simulink model "Step_12_TheEstimatedINVDynamicsMatricesCTC"  (R2020a)
settings: Solver=ode4  StartTime=0.0  StopTime=10  FixedStep=2e-3  RelTol=1e-3
model workspace (MATLAB code in the model file):
  | dhparams = [0   0   0.6   0;
  |             0   0   0     pi/2;
  |             0   0   0.5   0];
  | 
  | rrrRobot = rigidBodyTree('DataFormat', 'column', 'MaxNumBodies', 4);
  | 
  | bodyNames = {'link1', 'link2', 'link3'};
  | jointNames = {'joint1', 'joint2', 'joint3'};
  | parentNames = {'base', 'link1', 'link2'};
  | 
  | for i = 1:3
  |     body = rigidBody(bodyNames{i});
  |     joint = rigidBodyJoint(jointNames{i}, 'revolute');
  |     setFixedTransform(joint, dhparams(i,:), 'dh');
  |     body.Joint = joint;
  |     addBody(rrrRobot, body, parentNames{i});
  | end
  | 
  | tool = rigidBody('tool');
  | jointTool = rigidBodyJoint('fix_tip', 'fixed');
  | setFixedTransform(jointTool, eye(4));
  | tool.Joint = jointTool;
  | addBody(rrrRobot, tool, 'link3');
values from neighbouring files (symbols this model uses):
  N = simplify(N,'Seconds',30)    [Step_1_GetTheRegressorMatrix.m]    (also in Step_1_TheRegressorModel.m)
  s = size(M)    [Step_1_GetTheRegressorMatrix.m]    (also in Step_1_TheRegressorModel.m)
  Y = sym(zeros(robot.nbDOF,numel(Xhi)))    [Step_1_GetTheRegressorMatrix.m]    (also in Step_1_TheRegressorModel.m)
  Z = robot.symbolicParameters.Z    [Step_1_GetTheRegressorMatrix.m]    (also in Step_1_TheRegressorModel.m)
undefined symbols (not defined in the file or in its folder): X
libraries: sm_lib x34, nesl_utility x10
(part 2 of 2)

== matlab function Step_12_TheEstimatedINVDynamicsMatricesCTC/CTC/Estimated_C ==
  data: in1 input; EstTau_C output; in2 input
function EstTau_C = Estimated_C(in1,in2)
%#codegen

%    This function was generated by the Symbolic Math Toolbox version 8.5.
%    15-Jul-2026 04:23:10

q1 = in1(1,:);
q2 = in1(2,:);
q3 = in1(3,:);
qp1 = in2(1,:);
qp2 = in2(2,:);
qp3 = in2(3,:);
EstTau_C = [qp1.*2.995651003090984e-1+tanh(qp1.*1.0e+2).*2.011490037900599e-1+(cos(q2+q3).*cos(q1).*(qp2.*cos(q1)+qp3.*cos(q1))+cos(q2+q3).*sin(q1).*(qp2.*sin(q1)+qp3.*sin(q1))).*(qp1.*sin(q2+q3)-cos(q2+q3).*sin(q1).*(qp2.*cos(q1)+qp3.*cos(q1))+cos(q2+q3).*cos(q1).*(qp2.*sin(q1)+qp3.*sin(q1))).*1.461022037882879e-2+cos(q2+q3).*(sin(q1).*(qp1.*qp2.*cos(q1)+qp1.*qp3.*cos(q1))-cos(q1).*(qp1.*qp2.*sin(q1)+qp1.*qp3.*sin(q1))).*8.257807196549019e-4+(qp2.*cos(q1).^2.*sin(q2)+qp2.*sin(q1).^2.*sin(q2)).*(qp2.*cos(q1).^2+qp2.*sin(q1).^2).*1.019521576964412e-3-(cos(q2+q3).*cos(q1).*(qp2.*cos(q1)+qp3.*cos(q1))+cos(q2+q3).*sin(q1).*(qp2.*sin(q1)+qp3.*sin(q1))).*(qp1.*cos(q2+q3)+sin(q2+q3).*sin(q1).*(qp2.*cos(q1)+qp3.*cos(q1))-sin(q2+q3).*cos(q1).*(qp2.*sin(q1)+qp3.*sin(q1))).*4.225263872871405e-4-sin(q2+q3).*(sin(q1).*(qp1.*qp2.*cos(q1)+qp1.*qp3.*cos(q1))-cos(q1).*(qp1.*qp2.*sin(q1)+qp1.*qp3.*sin(q1))).*4.587581372374521e-4+(sin(q2+q3).*cos(q1).*(qp2.*cos(q1)+qp3.*cos(q1))+sin(q2+q3).*sin(q1).*(qp2.*sin(q1)+qp3.*sin(q1))).*(qp1.*sin(q2+q3)-cos(q2+q3).*sin(q1).*(qp2.*cos(q1)+qp3.*cos(q1))+cos(q2+q3).*cos(q1).*(qp2.*sin(q1)+qp3.*sin(q1))).*4.225263872871405e-4-cos(q2+q3).*((cos(q1).*cos(q2).*(qp1.*qp2.*cos(q1)+qp1.*qp3.*cos(q1)))./2.0+(cos(q2).*sin(q1).*(qp1.*qp2.*sin(q1)+qp1.*qp3.*sin(q1)))./2.0+(qp1.*cos(q1).*cos(q2).*(qp2.*cos(q1)+qp3.*cos(q1)))./2.0+(qp1.*cos(q2).*sin(q1).*(qp2.*sin(q1)+qp3.*sin(q1)))./2.0).*2.255824778756872e-3+cos(q2).*(qp1.*qp2.*cos(q1).^2.*cos(q2)+qp1.*qp2.*cos(q2).*sin(q1).^2).*1.124368820605591e-3-(sin(q2+q3).*cos(q1).*(qp2.*cos(q1)+qp3.*cos(q1))+sin(q2+q3).*sin(q1).*(qp2.*sin(q1)+qp3.*sin(q1))).*(qp1.*cos(q2+q3)+sin(q2+q3).*sin(q1).*(qp2.*cos(q1)+qp3.*cos(q1))-sin(q2+q3).*cos(q1).*(qp2.*sin(q1)+qp3.*sin(q1))).*9.399293254739789e-2-(sin(q1).*(qp2.*sin(q1)+qp3.*sin(q1))+cos(q1).*(qp2.*cos(q1)+qp3.*cos(q1))).*(cos(q2+q3).*cos(q1).*(qp2.*cos(q1)+qp3.*cos(q1))+cos(q2+q3).*sin(q1).*(qp2.*sin(q1)+qp3.*sin(q1))).*4.587581372374521e-4-sin(q2+q3).*((cos(q1).*cos(q2).*(qp1.*qp2.*cos(q1)+qp1.*qp3.*cos(q1)))./2.0+(cos(q2).*sin(q1).*(qp1.*qp2.*sin(q1)+qp1.*qp3.*sin(q1)))./2.0+(qp1.*cos(q1).*cos(q2).*(qp2.*cos(q1)+qp3.*cos(q1)))./2.0+(qp1.*cos(q2).*sin(q1).*(qp2.*sin(q1)+qp3.*sin(q1)))./2.0).*2.999511617512276e-1-cos(q2).*(qp1.*qp2.*cos(q1).^2.*sin(q2)+qp1.*qp2.*sin(q1).^2.*sin(q2)).*5.841025348904085e-1-cos(q2+q3).*(cos(q2+q3).*cos(q1).*(qp1.*qp2.*cos(q1)+qp1.*qp3.*cos(q1))+cos(q2+q3).*sin(q1).*(qp1.*qp2.*sin(q1)+qp1.*qp3.*sin(q1))).*4.225263872871405e-4-(sin(q1).*(qp2.*sin(q1)+qp3.*sin(q1))+cos(q1).*(qp2.*cos(q1)+qp3.*cos(q1))).*(sin(q2+q3).*cos(q1).*(qp2.*cos(q1)+qp3.*cos(q1))+sin(q2+q3).*sin(q1).*(qp2.*sin(q1)+qp3.*sin(q1))).*8.257807196549019e-4-sin(q2).*(qp1.*qp2.*cos(q1).^2.*sin(q2)+qp1.*qp2.*sin(q1).^2.*sin(q2)).*1.124368820605591e-3+sin(q2+q3).*(cos(q2+q3).*cos(q1).*(qp1.*qp2.*cos(q1)+qp1.*qp3.*cos(q1))+cos(q2+q3).*sin(q1).*(qp1.*qp2.*sin(q1)+qp1.*qp3.*sin(q1))).*1.461022037882879e-2-cos(q2+q3).*(sin(q2+q3).*cos(q1).*(qp1.*qp2.*cos(q1)+qp1.*qp3.*cos(q1))+sin(q2+q3).*sin(q1).*(qp1.*qp2.*sin(q1)+qp1.*qp3.*sin(q1))).*9.399293254739789e-2+sin(q2+q3).*(sin(q2+q3).*cos(q1).*(qp1.*qp2.*cos(q1)+qp1.*qp3.*cos(q1))+sin(q2+q3).*sin(q1).*(qp1.*qp2.*sin(q1)+qp1.*qp3.*sin(q1))).*4.225263872871405e-4-(sin(q1).*(qp2.*cos(q1)+qp3.*cos(q1))-cos(q1).*(qp2.*sin(q1)+qp3.*sin(q1))).*(qp1.*sin(q2+q3)-cos(q2+q3).*sin(q1).*(qp2.*cos(q1)+qp3.*cos(q1))+cos(q2+q3).*cos(q1).*(qp2.*sin(q1)+qp3.*sin(q1))).*4.587581372374521e-4+(sin(q1).*(qp2.*cos(q1)+qp3.*cos(q1))-cos(q1).*(qp2.*sin(q1)+qp3.*sin(q1))).*(qp1.*cos(q2+q3)+sin(q2+q3).*sin(q1).*(qp2.*cos(q1)+qp3.*cos(q1))-sin(q2+q3).*cos(q1).*(qp2.*sin(q1)+qp3.*sin(q1))).*8.257807196549019e-4+(sin(q1).*(qp2.*sin(q1)+qp3.*sin(q1))+cos(q1).*(qp2.*cos(q1)+qp3.*cos(q1))).*(sin(q1).*(qp2.*cos(q1)+qp3.*cos(q1))-cos(q1).*(qp2.*sin(q1)+qp3.*sin(q1))).*8.392301883660855e-2+(qp2.*cos(q1).^2.*cos(q2)+qp2.*cos(q2).*sin(q1).^2).*(qp2.*cos(q1).^2+qp2.*sin(q1).^2).*1.026288799911739e-3-cos(q2+q3).*cos(q1).*(qp1.*((qp1.*cos(q2).*sin(q1))./2.0+(qp2.*cos(q1).*sin(q2))./2.0)+qp2.*((qp1.*cos(q1).*sin(q2))./2.0+(qp2.*cos(q2).*sin(q1))./2.0)-(qp2.*cos(q1)+qp3.*cos(q1)).*((cos(q2).*sin(q1).*(qp2.*cos(q1)+qp3.*cos(q1)))./2.0-(cos(q1).*cos(q2).*(qp2.*sin(q1)+qp3.*sin(q1)))./2.0)-(qp1.^2.*cos(q2).*sin(q1))./2.0).*2.999511617512276e-1+sin(q2+q3).*cos(q1).*(qp1.*((qp1.*cos(q2).*sin(q1))./2.0+(qp2.*cos(q1).*sin(q2))./2.0)+qp2.*((qp1.*cos(q1).*sin(q2))./2.0+(qp2.*cos(q2).*sin(q1))./2.0)-(qp2.*cos(q1)+qp3.*cos(q1)).*((cos(q2).*sin(q1).*(qp2.*cos(q1)+qp3.*cos(q1)))./2.0-(cos(q1).*cos(q2).*(qp2.*sin(q1)+qp3.*sin(q1)))./2.0)-(qp1.^2.*cos(q2).*sin(q1))./2.0).*2.255824778756872e-3+cos(q2+q3).*sin(q1).*((qp2.*sin(q1)+qp3.*sin(q1)).*((cos(q2).*sin(q1).*(qp2.*cos(q1)+qp3.*cos(q1)))./2.0-(cos(q1).*cos(q2).*(qp2.*sin(q1)+qp3.*sin(q1)))./2.0)+qp1.*((qp1.*cos(q1).*cos(q2))./2.0-(qp2.*sin(q1).*sin(q2))./2.0)+qp2.*((qp2.*cos(q1).*cos(q2))./2.0-(qp1.*sin(q1).*sin(q2))./2.0)-(qp1.^2.*cos(q1).*cos(q2))./2.0).*2.999511617512276e-1+qp1.*cos(q2).*(qp2.*cos(q1).^2.*cos(q2)+qp2.*cos(q2).*sin(q1).^2).*1.124368820605591e-3-sin(q2+q3).*sin(q1).*((qp2.*sin(q1)+qp3.*sin(q1)).*((cos(q2).*sin(q1).*(qp2.*cos(q1)+qp3.*cos(q1)))./2.0-(cos(q1).*cos(q2).*(qp2.*sin(q1)+qp3.*sin(q1)))./2.0)+qp1.*((qp1.*cos(q1).*cos(q2))./2.0-(qp2.*sin(q1).*sin(q2))./2.0)+qp2.*((qp2.*cos(q1).*cos(q2))./2.0-(qp1.*sin(q1).*sin(q2))./2.0)-(qp1.^2.*cos(q1).*cos(q2))./2.0).*2.255824778756872e-3-qp1.*cos(q2).*(qp2.*cos(q1).^2.*sin(q2)+qp2.*sin(q1).^2.*sin(q2)).*5.841025348904085e-1-qp1.*sin(q2).*(qp2.*cos(q1).^2.*sin(q2)+qp2.*sin(q1).^2.*sin(q2)).*1.124368820605591e-3;qp2.*6.044333007850473e-1+tanh(qp2.*1.0e+2).*4.92616612948365e-1-sin(q1).*((cos(q2+q3).*(qp2.*cos(q1)+qp3.*cos(q1))-qp1.*sin(q2+q3).*sin(q1)).*(qp1.*cos(q2+q3)+sin(q2+q3).*sin(q1).*(qp2.*cos(q1)+qp3.*cos(q1))-sin(q2+q3).*cos(q1).*(qp2.*sin(q1)+qp3.*sin(q1)))-sin(q2+q3).*cos(q1).*(sin(q2+q3).*cos(q1).*(qp1.*qp2.*cos(q1)+qp1.*qp3.*cos(q1))+sin(q2+q3).*sin(q1).*(qp1.*qp2.*sin(q1)+qp1.*qp3.*sin(q1)))).*9.399293254739789e-2-sin(q1).*(-(sin(q1).*(qp2.*sin(q1)+qp3.*sin(q1))+cos(q1).*(qp2.*cos(q1)+qp3.*cos(q1))).*(sin(q2+q3).*(qp2.*cos(q1)+qp3.*cos(q1))+qp1.*cos(q2+q3).*sin(q1))+sin(q1).*(cos(q2+q3).*cos(q1).*(qp1.*qp2.*cos(q1)+qp1.*qp3.*cos(q1))+cos(q2+q3).*sin(q1).*(qp1.*qp2.*sin(q1)+qp1.*qp3.*sin(q1)))+qp1.*cos(q1).*(qp1.*sin(q2+q3)-cos(q2+q3).*sin(q1).*(qp2.*cos(q1)+qp3.*cos(q1))+cos(q2+q3).*cos(q1).*(qp2.*sin(q1)+qp3.*sin(q1)))+cos(q2+q3).*cos(q1).*(sin(q1).*(qp1.*qp2.*cos(q1)+qp1.*qp3.*cos(q1))-cos(q1).*(qp1.*qp2.*sin(q1)+qp1.*qp3.*sin(q1)))).*4.587581372374521e-4-cos(q1).*(-cos(q1).*(qp1.*qp2.*cos(q1).^2.*cos(q2)+qp1.*qp2.*cos(q2).*sin(q1).^2)+(qp1.*cos(q1).*cos(q2)-qp2.*sin(q1).*sin(q2)).*(qp2.*cos(q1).^2+qp2.*sin(q1).^2)+qp1.^2.*sin(q1).*sin(q2)).*1.026288799911739e-3-cos(q2+q3).*((qp2.*sin(q1)+qp3.*sin(q1)).*((cos(q2).*(qp2.*sin(q1)+qp3.*sin(q1)))./2.0+(qp1.*cos(q1).*sin(q2))./2.0)-cos(q1).*(qp1.*((qp1.*cos(q1).*cos(q2))./2.0-(qp2.*sin(q1).*sin(q2))./2.0)+qp2.*((qp2.*cos(q1).*cos(q2))./2.0-(qp1.*sin(q1).*sin(q2))./2.0))-sin(q1).*(qp1.*((qp1.*cos(q2).*sin(q1))./2.0+(qp2.*cos(q1).*sin(q2))./2.0)+qp2.*((qp1.*cos(q1).*sin(q2))./2.0+(qp2.*cos(q2).*sin(q1))./2.0))+(qp2.*cos(q1)+qp3.*cos(q1)).*((cos(q2).*(qp2.*cos(q1)+qp3.*cos(q1)))./2.0-(qp1.*sin(q1).*sin(q2))./2.0)-(sin(q1).*sin(q2).*(qp1.*qp2.*cos(q1)+qp1.*qp3.*cos(q1)))./2.0+(cos(q1).*sin(q2).*(qp1.*qp2.*sin(q1)+qp1.*qp3.*sin(q1)))./2.0).*2.255824778756872e-3+cos(q1).*((cos(q2+q3).*(qp2.*sin(q1)+qp3.*sin(q1))+qp1.*sin(q2+q3).*cos(q1)).*(qp1.*cos(q2+q3)+sin(q2+q3).*sin(q1).*(qp2.*cos(q1)+qp3.*cos(q1))-sin(q2+q3).*cos(q1).*(qp2.*sin(q1)+qp3.*sin(q1)))-sin(q2+q3).*sin(q1).*(sin(q2+q3).*cos(q1).*(qp1.*qp2.*cos(q1)+qp1.*qp3.*cos(q1))+sin(q2+q3).*sin(q1).*(qp1.*qp2.*sin(q1)+qp1.*qp3.*sin(q1)))).*9.399293254739789e-2-cos(q1).*((sin(q1).*(qp2.*sin(q1)+qp3.*sin(q1))+cos(q1).*(qp2.*cos(q1)+qp3.*cos(q1))).*(sin(q2+q3).*(qp2.*sin(q1)+qp3.*sin(q1))-qp1.*cos(q2+q3).*cos(q1))+cos(q1).*(cos(q2+q3).*cos(q1).*(qp1.*qp2.*cos(q1)+qp1.*qp3.*cos(q1))+cos(q2+q3).*sin(q1).*(qp1.*qp2.*sin(q1)+qp1.*qp3.*sin(q1)))-qp1.*sin(q1).*(qp1.*sin(q2+q3)-cos(q2+q3).*sin(q1).*(qp2.*cos(q1)+qp3.*cos(q1))+cos(q2+q3).*cos(q1).*(qp2.*sin(q1)+qp3.*sin(q1)))-cos(q2+q3).*sin(q1).*(sin(q1).*(qp1.*qp2.*cos(q1)+qp1.*qp3.*cos(q1))-cos(q1).*(qp1.*qp2.*sin(q1)+qp1.*qp3.*sin(q1)))).*4.587581372374521e-4+cos(q1).*(-(qp1.*cos(q1).*sin(q2)+qp2.*cos(q2).*sin(q1)).*(qp2.*cos(q1).^2+qp2.*sin(q1).^2)+cos(q1).*(qp1.*qp2.*cos(q1).^2.*sin(q2)+qp1.*qp2.*sin(q1).^2.*sin(q2))+qp1.^2.*cos(q2).*sin(q1)).*1.019521576964412e-3+sin(q1).*(sin(q1).*(qp1.*qp2.*cos(q1).^2.*cos(q2)+qp1.*qp2.*cos(q2).*sin(q1).^2)-(qp1.*cos(q2).*sin(q1)+qp2.*cos(q1).*sin(q2)).*(qp2.*cos(q1).^2+qp2.*sin(q1).^2)+qp1.^2.*cos(q1).*sin(q2)).*1.026288799911739e-3-sin(q2+q3).*((qp2.*sin(q1)+qp3.*sin(q1)).*((cos(q2).*(qp2.*sin(q1)+qp3.*sin(q1)))./2.0+(qp1.*cos(q1).*sin(q2))./2.0)-cos(q1).*(qp1.*((qp1.*cos(q1).*cos(q2))./2.0-(qp2.*sin(q1).*sin(q2))./2.0)+qp2.*((qp2.*cos(q1).*cos(q2))./2.0-(qp1.*sin(q1).*sin(q2))./2.0))-sin(q1).*(qp1.*((qp1.*cos(q2).*sin(q1))./2.0+(qp2.*cos(q1).*sin(q2))./2.0)+qp2.*((qp1.*cos(q1).*sin(q2))./2.0+(qp2.*cos(q2).*sin(q1))./2.0))+(qp2.*cos(q1)+qp3.*cos(q1)).*((cos(q2).*(qp2.*cos(q1)+qp3.*cos(q1)))./2.0-(qp1.*sin(q1).*sin(q2))./2.0)-(sin(q1).*sin(q2).*(qp1.*qp2.*cos(q1)+qp1.*qp3.*cos(q1)))./2.0+(cos(q1).*sin(q2).*(qp1.*qp2.*sin(q1)+qp1.*qp3.*sin(q1)))./2.0).*2.999511617512276e-1-sin(q1).*(qp1.*cos(q2).*(qp1.*cos(q2).*sin(q1)+qp2.*cos(q1).*sin(q2))+cos(q1).*sin(q2).*(qp1.*qp2.*cos(q1).^2.*cos(q2)+qp1.*qp2.*cos(q2).*sin(q1).^2)+qp1.*sin(q2).*(qp2.*cos(q1).*cos(q2)-qp1.*sin(q1).*sin(q2))+cos(q1).*cos(q2).*(qp1.*qp2.*cos(q1).^2.*sin(q2)+qp1.*qp2.*sin(q1).^2.*sin(q2))).*1.124368820605591e-3+sin(q1).*((sin(q2+q3).*(qp2.*cos(q1)+qp3.*cos(q1))+qp1.*cos(q2+q3).*sin(q1)).*(qp1.*cos(q2+q3)+sin(q2+q3).*sin(q1).*(qp2.*cos(q1)+qp3.*cos(q1))-sin(q2+q3).*cos(q1).*(qp2.*sin(q1)+qp3.*sin(q1)))+(cos(q2+q3).*(qp2.*cos(q1)+qp3.*cos(q1))-qp1.*sin(q2+q3).*sin(q1)).*(qp1.*sin(q2+q3)-cos(q2+q3).*sin(q1).*(qp2.*cos(q1)+qp3.*cos(q1))+cos(q2+q3).*cos(q1).*(qp2.*sin(q1)+qp3.*sin(q1)))+sin(q2+q3).*cos(q1).*(cos(q2+q3).*cos(q1).*(qp1.*qp2.*cos(q1)+qp1.*qp3.*cos(q1))+cos(q2+q3).*sin(q1).*(qp1.*qp2.*sin(q1)+qp1.*qp3.*sin(q1)))+cos(q2+q3).*cos(q1).*(sin(q2+q3).*cos(q1).*(qp1.*qp2.*cos(q1)+qp1.*qp3.*cos(q1))+sin(q2+q3).*sin(q1).*(qp1.*qp2.*sin(q1)+qp1.*qp3.*sin(q1)))).*4.225263872871405e-4+sin(q1).*((qp2.*cos(q1).*cos(q2)-qp1.*sin(q1).*sin(q2)).*(qp2.*cos(q1).^2+qp2.*sin(q1).^2)+sin(q1).*(qp1.*qp2.*cos(q1).^2.*sin(q2)+qp1.*qp2.*sin(q1).^2.*sin(q2))-qp1.^2.*cos(q1).*cos(q2)).*1.019521576964412e-3+cos(q2+q3).*cos(q1).^2.*2.93952138516203+cos(q1).*(-qp1.*cos(q2).*(qp1.*cos(q1).*cos(q2)-qp2.*sin(q1).*sin(q2))+qp1.*sin(q2).*(qp1.*cos(q1).*sin(q2)+qp2.*cos(q2).*sin(q1))+sin(q1).*sin(q2).*(qp1.*qp2.*cos(q1).^2.*cos(q2)+qp1.*qp2.*cos(q2).*sin(q1).^2)+cos(q2).*sin(q1).*(qp1.*qp2.*cos(q1).^2.*sin(q2)+qp1.*qp2.*sin(q1).^2.*sin(q2))).*1.124368820605591e-3+cos(q2+q3).*sin(q1).^2.*2.93952138516203-sin(q2+q3).*cos(q1).^2.*2.210708283181735e-2-sin(q1).*((sin(q1).*(qp2.*sin(q1)+qp3.*sin(q1))+cos(q1).*(qp2.*cos(q1)+qp3.*cos(q1))).*(cos(q2+q3).*(qp2.*cos(q1)+qp3.*cos(q1))-qp1.*sin(q2+q3).*sin(q1))+sin(q1).*(sin(q2+q3).*cos(q1).*(qp1.*qp2.*cos(q1)+qp1.*qp3.*cos(q1))+sin(q2+q3).*sin(q1).*(qp1.*qp2.*sin(q1)+qp1.*qp3.*sin(q1)))-qp1.*cos(q1).*(qp1.*cos(q2+q3)+sin(q2+q3).*sin(q1).*(qp2.*cos(q1)+qp3.*cos(q1))-sin(q2+q3).*cos(q1).*(qp2.*sin(q1)+qp3.*sin(q1)))+sin(q2+q3).*cos(q1).*(sin(q1).*(qp1.*qp2.*cos(q1)+qp1.*qp3.*cos(q1))-cos(q1).*(qp1.*qp2.*sin(q1)+qp1.*qp3.*sin(q1)))).*8.257807196549019e-4-sin(q2+q3).*sin(q1).^2.*2.210708283181735e-2+cos(q1).*((sin(q1).*(qp2.*sin(q1)+qp3.*sin(q1))+cos(q1).*(qp2.*cos(q1)+qp3.*cos(q1))).*(cos(q2+q3).*(qp2.*sin(q1)+qp3.*sin(q1))+qp1.*sin(q2+q3).*cos(q1))-cos(q1).*(sin(q2+q3).*cos(q1).*(qp1.*qp2.*cos(q1)+qp1.*qp3.*cos(q1))+sin(q2+q3).*sin(q1).*(qp1.*qp2.*sin(q1)+qp1.*qp3.*sin(q1)))+sin(q2+q3).*sin(q1).*(sin(q1).*(qp1.*qp2.*cos(q1)+qp1.*qp3.*cos(q1))-cos(q1).*(qp1.*qp2.*sin(q1)+qp1.*qp3.*sin(q1)))-qp1.*sin(q1).*(qp1.*cos(q2+q3)+sin(q2+q3).*sin(q1).*(qp2.*cos(q1)+qp3.*cos(q1))-sin(q2+q3).*cos(q1).*(qp2.*sin(q1)+qp3.*sin(q1)))).*8.257807196549019e-4-cos(q1).*((cos(q2+q3).*(qp2.*sin(q1)+qp3.*sin(q1))+qp1.*sin(q2+q3).*cos(q1)).*(qp1.*sin(q2+q3)-cos(q2+q3).*sin(q1).*(qp2.*cos(q1)+qp3.*cos(q1))+cos(q2+q3).*cos(q1).*(qp2.*sin(q1)+qp3.*sin(q1)))+(sin(q2+q3).*(qp2.*sin(q1)+qp3.*sin(q1))-qp1.*cos(q2+q3).*cos(q1)).*(qp1.*cos(q2+q3)+sin(q2+q3).*sin(q1).*(qp2.*cos(q1)+qp3.*cos(q1))-sin(q2+q3).*cos(q1).*(qp2.*sin(q1)+qp3.*sin(q1)))+sin(q2+q3).*sin(q1).*(cos(q2+q3).*cos(q1).*(qp1.*qp2.*cos(q1)+qp1.*qp3.*cos(q1))+cos(q2+q3).*sin(q1).*(qp1.*qp2.*sin(q1)+qp1.*qp3.*sin(q1)))+cos(q2+q3).*sin(q1).*(sin(q2+q3).*cos(q1).*(qp1.*qp2.*cos(q1)+qp1.*qp3.*cos(q1))+sin(q2+q3).*sin(q1).*(qp1.*qp2.*sin(q1)+qp1.*qp3.*sin(q1)))).*4.225263872871405e-4-sin(q1).*((sin(q2+q3).*(qp2.*cos(q1)+qp3.*cos(q1))+qp1.*cos(q2+q3).*sin(q1)).*(qp1.*sin(q2+q3)-cos(q2+q3).*sin(q1).*(qp2.*cos(q1)+qp3.*cos(q1))+cos(q2+q3).*cos(q1).*(qp2.*sin(q1)+qp3.*sin(q1)))-cos(q2+q3).*cos(q1).*(cos(q2+q3).*cos(q1).*(qp1.*qp2.*cos(q1)+qp1.*qp3.*cos(q1))+cos(q2+q3).*sin(q1).*(qp1.*qp2.*sin(q1)+qp1.*qp3.*sin(q1)))).*1.461022037882879e-2+cos(q1).*(cos(q1).*(sin(q1).*(qp1.*qp2.*cos(q1)+qp1.*qp3.*cos(q1))-cos(q1).*(qp1.*qp2.*sin(q1)+qp1.*qp3.*sin(q1)))-qp1.*sin(q1).*(sin(q1).*(qp2.*sin(q1)+qp3.*sin(q1))+cos(q1).*(qp2.*cos(q1)+qp3.*cos(q1)))).*8.392301883660855e-2+cos(q1).*((sin(q2+q3).*(qp2.*sin(q1)+qp3.*sin(q1))-qp1.*cos(q2+q3).*cos(q1)).*(qp1.*sin(q2+q3)-cos(q2+q3).*sin(q1).*(qp2.*cos(q1)+qp3.*cos(q1))+cos(q2+q3).*cos(q1).*(qp2.*sin(q1)+qp3.*sin(q1)))-cos(q2+q3).*sin(q1).*(cos(q2+q3).*cos(q1).*(qp1.*qp2.*cos(q1)+qp1.*qp3.*cos(q1))+cos(q2+q3).*sin(q1).*(qp1.*qp2.*sin(q1)+qp1.*qp3.*sin(q1)))).*1.461022037882879e-2+sin(q1).*(sin(q1).*(sin(q1).*(qp1.*qp2.*cos(q1)+qp1.*qp3.*cos(q1))-cos(q1).*(qp1.*qp2.*sin(q1)+qp1.*qp3.*sin(q1)))+qp1.*cos(q1).*(sin(q1).*(qp2.*sin(q1)+qp3.*sin(q1))+cos(q1).*(qp2.*cos(q1)+qp3.*cos(q1)))).*8.392301883660855e-2+cos(q1).*(qp1.*cos(q2).*(qp1.*cos(q1).*sin(q2)+qp2.*cos(q2).*sin(q1))-sin(q1).*sin(q2).*(qp1.*qp2.*cos(q1).^2.*sin(q2)+qp1.*qp2.*sin(q1).^2.*sin(q2))).*5.841025348904085e-1-sin(q1).*(qp1.*cos(q2).*(qp2.*cos(q1).*cos(q2)-qp1.*sin(q1).*sin(q2))-cos(q1).*sin(q2).*(qp1.*qp2.*cos(q1).^2.*sin(q2)+qp1.*qp2.*sin(q1).^2.*sin(q2))).*5.841025348904085e-1+cos(q2+q3).*cos(q1).*(((cos(q1).*sin(q2).*(qp2.*cos(q1)+qp3.*cos(q1)))./2.0+(sin(q1).*sin(q2).*(qp2.*sin(q1)+qp3.*sin(q1)))./2.0).*(qp2.*cos(q1)+qp3.*cos(q1))-cos(q1).*((qp2.^2.*sin(q2))./2.0+4.9e+1./5.0)+qp1.*((cos(q2).*(qp2.*sin(q1)+qp3.*sin(q1)))./2.0+(qp1.*cos(q1).*sin(q2))./2.0)-(cos(q2).*(qp1.*qp2.*sin(q1)+qp1.*qp3.*sin(q1)))./2.0).*2.999511617512276e-1-sin(q2+q3).*cos(q1).*(((cos(q1).*sin(q2).*(qp2.*cos(q1)+qp3.*cos(q1)))./2.0+(sin(q1).*sin(q2).*(qp2.*sin(q1)+qp3.*sin(q1)))./2.0).*(qp2.*cos(q1)+qp3.*cos(q1))-cos(q1).*((qp2.^2.*sin(q2))./2.0+4.9e+1./5.0)+qp1.*((cos(q2).*(qp2.*sin(q1)+qp3.*sin(q1)))./2.0+(qp1.*cos(q1).*sin(q2))./2.0)-(cos(q2).*(qp1.*qp2.*sin(q1)+qp1.*qp3.*sin(q1)))./2.0).*2.255824778756872e-3+cos(q2+q3).*sin(q1).*(((cos(q1).*sin(q2).*(qp2.*cos(q1)+qp3.*cos(q1)))./2.0+(sin(q1).*sin(q2).*(qp2.*sin(q1)+qp3.*sin(q1)))./2.0).*(qp2.*sin(q1)+qp3.*sin(q1))-qp1.*((cos(q2).*(qp2.*cos(q1)+qp3.*cos(q1)))./2.0-(qp1.*sin(q1).*sin(q2))./2.0)-sin(q1).*((qp2.^2.*sin(q2))./2.0+4.9e+1./5.0)+(cos(q2).*(qp1.*qp2.*cos(q1)+qp1.*qp3.*cos(q1)))./2.0).*2.999511617512276e-1-sin(q2+q3).*sin(q1).*(((cos(q1).*sin(q2).*(qp2.*cos(q1)+qp3.*cos(q1)))./2.0+(sin(q1).*sin(q2).*(qp2.*sin(q1)+qp3.*sin(q1)))./2.0).*(qp2.*sin(q1)+qp3.*sin(q1))-qp1.*((cos(q2).*(qp2.*cos(q1)+qp3.*cos(q1)))./2.0-(qp1.*sin(q1).*sin(q2))./2.0)-sin(q1).*((qp2.^2.*sin(q2))./2.0+4.9e+1./5.0)+(cos(q2).*(qp1.*qp2.*cos(q1)+qp1.*qp3.*cos(q1)))./2.0).*2.255824778756872e-3;qp3.*5.444152870511105e-1+tanh(qp3.*1.0e+2).*7.756228967740465e-1-sin(q1).*((cos(q2+q3).*(qp2.*cos(q1)+qp3.*cos(q1))-qp1.*sin(q2+q3).*sin(q1)).*(qp1.*cos(q2+q3)+sin(q2+q3).*sin(q1).*(qp2.*cos(q1)+qp3.*cos(q1))-sin(q2+q3).*cos(q1).*(qp2.*sin(q1)+qp3.*sin(q1)))-sin(q2+q3).*cos(q1).*(sin(q2+q3).*cos(q1).*(qp1.*qp2.*cos(q1)+qp1.*qp3.*cos(q1))+sin(q2+q3).*sin(q1).*(qp1.*qp2.*sin(q1)+qp1.*qp3.*sin(q1)))).*9.399293254739789e-2-sin(q1).*(-(sin(q1).*(qp2.*sin(q1)+qp3.*sin(q1))+cos(q1).*(qp2.*cos(q1)+qp3.*cos(q1))).*(sin(q2+q3).*(qp2.*cos(q1)+qp3.*cos(q1))+qp1.*cos(q2+q3).*sin(q1))+sin(q1).*(cos(q2+q3).*cos(q1).*(qp1.*qp2.*cos(q1)+qp1.*qp3.*cos(q1))+cos(q2+q3).*sin(q1).*(qp1.*qp2.*sin(q1)+qp1.*qp3.*sin(q1)))+qp1.*cos(q1).*(qp1.*sin(q2+q3)-cos(q2+q3).*sin(q1).*(qp2.*cos(q1)+qp3.*cos(q1))+cos(q2+q3).*cos(q1).*(qp2.*sin(q1)+qp3.*sin(q1)))+cos(q2+q3).*cos(q1).*(sin(q1).*(qp1.*qp2.*cos(q1)+qp1.*qp3.*cos(q1))-cos(q1).*(qp1.*qp2.*sin(q1)+qp1.*qp3.*sin(q1)))).*4.587581372374521e-4+cos(q1).*((cos(q2+q3).*(qp2.*sin(q1)+qp3.*sin(q1))+qp1.*sin(q2+q3).*cos(q1)).*(qp1.*cos(q2+q3)+sin(q2+q3).*sin(q1).*(qp2.*cos(q1)+qp3.*cos(q1))-sin(q2+q3).*cos(q1).*(qp2.*sin(q1)+qp3.*sin(q1)))-sin(q2+q3).*sin(q1).*(sin(q2+q3).*cos(q1).*(qp1.*qp2.*cos(q1)+qp1.*qp3.*cos(q1))+sin(q2+q3).*sin(q1).*(qp1.*qp2.*sin(q1)+qp1.*qp3.*sin(q1)))).*9.399293254739789e-2-cos(q1).*((sin(q1).*(qp2.*sin(q1)+qp3.*sin(q1))+cos(q1).*(qp2.*cos(q1)+qp3.*cos(q1))).*(sin(q2+q3).*(qp2.*sin(q1)+qp3.*sin(q1))-qp1.*cos(q2+q3).*cos(q1))+cos(q1).*(cos(q2+q3).*cos(q1).*(qp1.*qp2.*cos(q1)+qp1.*qp3.*cos(q1))+cos(q2+q3).*sin(q1).*(qp1.*qp2.*sin(q1)+qp1.*qp3.*sin(q1)))-qp1.*sin(q1).*(qp1.*sin(q2+q3)-cos(q2+q3).*sin(q1).*(qp2.*cos(q1)+qp3.*cos(q1))+cos(q2+q3).*cos(q1).*(qp2.*sin(q1)+qp3.*sin(q1)))-cos(q2+q3).*sin(q1).*(sin(q1).*(qp1.*qp2.*cos(q1)+qp1.*qp3.*cos(q1))-cos(q1).*(qp1.*qp2.*sin(q1)+qp1.*qp3.*sin(q1)))).*4.587581372374521e-4+sin(q1).*((sin(q2+q3).*(qp2.*cos(q1)+qp3.*cos(q1))+qp1.*cos(q2+q3).*sin(q1)).*(qp1.*cos(q2+q3)+sin(q2+q3).*sin(q1).*(qp2.*cos(q1)+qp3.*cos(q1))-sin(q2+q3).*cos(q1).*(qp2.*sin(q1)+qp3.*sin(q1)))+(cos(q2+q3).*(qp2.*cos(q1)+qp3.*cos(q1))-qp1.*sin(q2+q3).*sin(q1)).*(qp1.*sin(q2+q3)-cos(q2+q3).*sin(q1).*(qp2.*cos(q1)+qp3.*cos(q1))+cos(q2+q3).*cos(q1).*(qp2.*sin(q1)+qp3.*sin(q1)))+sin(q2+q3).*cos(q1).*(cos(q2+q3).*cos(q1).*(qp1.*qp2.*cos(q1)+qp1.*qp3.*cos(q1))+cos(q2+q3).*sin(q1).*(qp1.*qp2.*sin(q1)+qp1.*qp3.*sin(q1)))+cos(q2+q3).*cos(q1).*(sin(q2+q3).*cos(q1).*(qp1.*qp2.*cos(q1)+qp1.*qp3.*cos(q1))+sin(q2+q3).*sin(q1).*(qp1.*qp2.*sin(q1)+qp1.*qp3.*sin(q1)))).*4.225263872871405e-4+cos(q2+q3).*cos(q1).^2.*2.93952138516203+cos(q2+q3).*sin(q1).^2.*2.93952138516203-sin(q2+q3).*cos(q1).^2.*2.210708283181735e-2-sin(q1).*((sin(q1).*(qp2.*sin(q1)+qp3.*sin(q1))+cos(q1).*(qp2.*cos(q1)+qp3.*cos(q1))).*(cos(q2+q3).*(qp2.*cos(q1)+qp3.*cos(q1))-qp1.*sin(q2+q3).*sin(q1))+sin(q1).*(sin(q2+q3).*cos(q1).*(qp1.*qp2.*cos(q1)+qp1.*qp3.*cos(q1))+sin(q2+q3).*sin(q1).*(qp1.*qp2.*sin(q1)+qp1.*qp3.*sin(q1)))-qp1.*cos(q1).*(qp1.*cos(q2+q3)+sin(q2+q3).*sin(q1).*(qp2.*cos(q1)+qp3.*cos(q1))-sin(q2+q3).*cos(q1).*(qp2.*sin(q1)+qp3.*sin(q1)))+sin(q2+q3).*cos(q1).*(sin(q1).*(qp1.*qp2.*cos(q1)+qp1.*qp3.*cos(q1))-cos(q1).*(qp1.*qp2.*sin(q1)+qp1.*qp3.*sin(q1)))).*8.257807196549019e-4-sin(q2+q3).*sin(q1).^2.*2.210708283181735e-2+cos(q1).*((sin(q1).*(qp2.*sin(q1)+qp3.*sin(q1))+cos(q1).*(qp2.*cos(q1)+qp3.*cos(q1))).*(cos(q2+q3).*(qp2.*sin(q1)+qp3.*sin(q1))+qp1.*sin(q2+q3).*cos(q1))-cos(q1).*(sin(q2+q3).*cos(q1).*(qp1.*qp2.*cos(q1)+qp1.*qp3.*cos(q1))+sin(q2+q3).*sin(q1).*(qp1.*qp2.*sin(q1)+qp1.*qp3.*sin(q1)))+sin(q2+q3).*sin(q1).*(sin(q1).*(qp1.*qp2.*cos(q1)+qp1.*qp3.*cos(q1))-cos(q1).*(qp1.*qp2.*sin(q1)+qp1.*qp3.*sin(q1)))-qp1.*sin(q1).*(qp1.*cos(q2+q3)+sin(q2+q3).*sin(q1).*(qp2.*cos(q1)+qp3.*cos(q1))-sin(q2+q3).*cos(q1).*(qp2.*sin(q1)+qp3.*sin(q1)))).*8.257807196549019e-4-cos(q1).*((cos(q2+q3).*(qp2.*sin(q1)+qp3.*sin(q1))+qp1.*sin(q2+q3).*cos(q1)).*(qp1.*sin(q2+q3)-cos(q2+q3).*sin(q1).*(qp2.*cos(q1)+qp3.*cos(q1))+cos(q2+q3).*cos(q1).*(qp2.*sin(q1)+qp3.*sin(q1)))+(sin(q2+q3).*(qp2.*sin(q1)+qp3.*sin(q1))-qp1.*cos(q2+q3).*cos(q1)).*(qp1.*cos(q2+q3)+sin(q2+q3).*sin(q1).*(qp2.*cos(q1)+qp3.*cos(q1))-sin(q2+q3).*cos(q1).*(qp2.*sin(q1)+qp3.*sin(q1)))+sin(q2+q3).*sin(q1).*(cos(q2+q3).*cos(q1).*(qp1.*qp2.*cos(q1)+qp1.*qp3.*cos(q1))+cos(q2+q3).*sin(q1).*(qp1.*qp2.*sin(q1)+qp1.*qp3.*sin(q1)))+cos(q2+q3).*sin(q1).*(sin(q2+q3).*cos(q1).*(qp1.*qp2.*cos(q1)+qp1.*qp3.*cos(q1))+sin(q2+q3).*sin(q1).*(qp1.*qp2.*sin(q1)+qp1.*qp3.*sin(q1)))).*4.225263872871405e-4+cos(q2+q3).*(cos(q1).*(qp1.*((qp1.*cos(q1).*cos(q2))./2.0-(qp2.*sin(q1).*sin(q2))./2.0)+qp2.*((qp2.*cos(q1).*cos(q2))./2.0-(qp1.*sin(q1).*sin(q2))./2.0))+sin(q1).*(qp1.*((qp1.*cos(q2).*sin(q1))./2.0+(qp2.*cos(q1).*sin(q2))./2.0)+qp2.*((qp1.*cos(q1).*sin(q2))./2.0+(qp2.*cos(q2).*sin(q1))./2.0))).*2.255824778756872e-3+sin(q2+q3).*(cos(q1).*(qp1.*((qp1.*cos(q1).*cos(q2))./2.0-(qp2.*sin(q1).*sin(q2))./2.0)+qp2.*((qp2.*cos(q1).*cos(q2))./2.0-(qp1.*sin(q1).*sin(q2))./2.0))+sin(q1).*(qp1.*((qp1.*cos(q2).*sin(q1))./2.0+(qp2.*cos(q1).*sin(q2))./2.0)+qp2.*((qp1.*cos(q1).*sin(q2))./2.0+(qp2.*cos(q2).*sin(q1))./2.0))).*2.999511617512276e-1-sin(q1).*((sin(q2+q3).*(qp2.*cos(q1)+qp3.*cos(q1))+qp1.*cos(q2+q3).*sin(q1)).*(qp1.*sin(q2+q3)-cos(q2+q3).*sin(q1).*(qp2.*cos(q1)+qp3.*cos(q1))+cos(q2+q3).*cos(q1).*(qp2.*sin(q1)+qp3.*sin(q1)))-cos(q2+q3).*cos(q1).*(cos(q2+q3).*cos(q1).*(qp1.*qp2.*cos(q1)+qp1.*qp3.*cos(q1))+cos(q2+q3).*sin(q1).*(qp1.*qp2.*sin(q1)+qp1.*qp3.*sin(q1)))).*1.461022037882879e-2+cos(q1).*(cos(q1).*(sin(q1).*(qp1.*qp2.*cos(q1)+qp1.*qp3.*cos(q1))-cos(q1).*(qp1.*qp2.*sin(q1)+qp1.*qp3.*sin(q1)))-qp1.*sin(q1).*(sin(q1).*(qp2.*sin(q1)+qp3.*sin(q1))+cos(q1).*(qp2.*cos(q1)+qp3.*cos(q1)))).*8.392301883660855e-2+cos(q1).*((sin(q2+q3).*(qp2.*sin(q1)+qp3.*sin(q1))-qp1.*cos(q2+q3).*cos(q1)).*(qp1.*sin(q2+q3)-cos(q2+q3).*sin(q1).*(qp2.*cos(q1)+qp3.*cos(q1))+cos(q2+q3).*cos(q1).*(qp2.*sin(q1)+qp3.*sin(q1)))-cos(q2+q3).*sin(q1).*(cos(q2+q3).*cos(q1).*(qp1.*qp2.*cos(q1)+qp1.*qp3.*cos(q1))+cos(q2+q3).*sin(q1).*(qp1.*qp2.*sin(q1)+qp1.*qp3.*sin(q1)))).*1.461022037882879e-2+sin(q1).*(sin(q1).*(sin(q1).*(qp1.*qp2.*cos(q1)+qp1.*qp3.*cos(q1))-cos(q1).*(qp1.*qp2.*sin(q1)+qp1.*qp3.*sin(q1)))+qp1.*cos(q1).*(sin(q1).*(qp2.*sin(q1)+qp3.*sin(q1))+cos(q1).*(qp2.*cos(q1)+qp3.*cos(q1)))).*8.392301883660855e-2-cos(q2+q3).*cos(q1).^2.*((qp2.^2.*sin(q2))./2.0+4.9e+1./5.0).*2.999511617512276e-1-cos(q2+q3).*sin(q1).^2.*((qp2.^2.*sin(q2))./2.0+4.9e+1./5.0).*2.999511617512276e-1+sin(q2+q3).*cos(q1).^2.*((qp2.^2.*sin(q2))./2.0+4.9e+1./5.0).*2.255824778756872e-3+sin(q2+q3).*sin(q1).^2.*((qp2.^2.*sin(q2))./2.0+4.9e+1./5.0).*2.255824778756872e-3];

== matlab function Step_12_TheEstimatedINVDynamicsMatricesCTC/CTC/Estimated_G ==
  data: in1 input; EstTau_G output
function EstTau_G = Estimated_G(in1)
%#codegen

%    This function was generated by the Symbolic Math Toolbox version 8.5.
%    15-Jul-2026 04:23:10

q1 = in1(1,:);
q2 = in1(2,:);
q3 = in1(3,:);
EstTau_G = [0.0;cos(q2+q3).*cos(q1).^2.*(-2.93952138516203)-cos(q2+q3).*sin(q1).^2.*2.93952138516203+sin(q2+q3).*cos(q1).^2.*2.210708283181735e-2+sin(q2+q3).*sin(q1).^2.*2.210708283181735e-2-cos(q1).^2.*cos(q2).*1.348620116356317e+1-cos(q2).*sin(q1).^2.*1.348620116356317e+1+cos(q1).^2.*sin(q2).*3.617991560015852e-3+sin(q1).^2.*sin(q2).*3.617991560015852e-3;cos(q2+q3).*cos(q1).^2.*(-2.93952138516203)-cos(q2+q3).*sin(q1).^2.*2.93952138516203+sin(q2+q3).*cos(q1).^2.*2.210708283181735e-2+sin(q2+q3).*sin(q1).^2.*2.210708283181735e-2];

== matlab function Step_12_TheEstimatedINVDynamicsMatricesCTC/CTC/Estimated_M ==
  data: in1 input; EstTau_M output
function EstTau_M = Estimated_M(in1)
%#codegen

%    This function was generated by the Symbolic Math Toolbox version 8.5.
%    15-Jul-2026 04:23:10

q1 = in1(1,:);
q2 = in1(2,:);
q3 = in1(3,:);
EstTau_M = reshape([cos(q2+q3).^2.*9.399293254739789e-2+sin(q2+q3).^2.*1.461022037882879e-2+cos(q2).*sin(q2).*2.248737641211183e-3+cos(q2).^2.*5.841025348904085e-1-cos(q2+q3).*sin(q2+q3).*8.450527745742809e-4+cos(q2+q3).*cos(q1).^2.*cos(q2).*2.999511617512276e-1+cos(q2+q3).*cos(q2).*sin(q1).^2.*2.999511617512276e-1-sin(q2+q3).*cos(q1).^2.*cos(q2).*2.255824778756872e-3-sin(q2+q3).*cos(q2).*sin(q1).^2.*2.255824778756872e-3,sin(q1).*(cos(q2+q3).^2.*cos(q1)-sin(q2+q3).^2.*cos(q1)).*(-4.225263872871405e-4)+cos(q1).*(cos(q2+q3).^2.*sin(q1)-sin(q2+q3).^2.*sin(q1)).*4.225263872871405e-4+cos(q2+q3).*cos(q1).^2.*8.257807196549019e-4+cos(q2+q3).*sin(q1).^2.*8.257807196549019e-4-sin(q2+q3).*cos(q1).^2.*4.587581372374521e-4-sin(q2+q3).*sin(q1).^2.*4.587581372374521e-4-cos(q1).^2.*cos(q2).*1.019521576964412e-3-cos(q2).*sin(q1).^2.*1.019521576964412e-3+cos(q1).^2.*sin(q2).*1.026288799911739e-3+sin(q1).*(cos(q1).*cos(q2).^2-cos(q1).*sin(q2).^2).*1.124368820605591e-3+sin(q1).^2.*sin(q2).*1.026288799911739e-3-cos(q1).*(cos(q2).^2.*sin(q1)-sin(q1).*sin(q2).^2).*1.124368820605591e-3,sin(q1).*(cos(q2+q3).^2.*cos(q1)-sin(q2+q3).^2.*cos(q1)).*(-4.225263872871405e-4)+cos(q1).*(cos(q2+q3).^2.*sin(q1)-sin(q2+q3).^2.*sin(q1)).*4.225263872871405e-4+cos(q2+q3).*cos(q1).^2.*8.257807196549019e-4+cos(q2+q3).*sin(q1).^2.*8.257807196549019e-4-sin(q2+q3).*cos(q1).^2.*4.587581372374521e-4-sin(q2+q3).*sin(q1).^2.*4.587581372374521e-4,cos(q2).*(cos(q1).^2+sin(q1).^2).*(-1.019521576964412e-3)+sin(q2).*(cos(q1).^2+sin(q1).^2).*1.026288799911739e-3+cos(q2+q3).*(cos(q1).^2+sin(q1).^2).*8.257807196549019e-4-sin(q2+q3).*(cos(q1).^2+sin(q1).^2).*4.587581372374521e-4,cos(q2+q3).*(cos(q1).^2.*sin(q2)+sin(q1).^2.*sin(q2)).*2.255824778756872e-3+cos(q1).^2.*(cos(q1).^2+sin(q1).^2).*6.678014559782907e-1+sin(q2+q3).*(cos(q1).^2.*sin(q2)+sin(q1).^2.*sin(q2)).*2.999511617512276e-1+sin(q1).^2.*(cos(q1).^2+sin(q1).^2).*6.678014559782907e-1+cos(q2+q3).*cos(q1).^2.*cos(q2).*2.999511617512276e-1+cos(q2+q3).*cos(q2).*sin(q1).^2.*2.999511617512276e-1-sin(q2+q3).*cos(q1).^2.*cos(q2).*2.255824778756872e-3-sin(q2+q3).*cos(q2).*sin(q1).^2.*2.255824778756872e-3,cos(q2+q3).*((cos(q1).^2.*sin(q2))./2.0+(sin(q1).^2.*sin(q2))./2.0).*2.255824778756872e-3+cos(q1).^2.*(cos(q1).^2+sin(q1).^2).*8.392301883660855e-2+sin(q2+q3).*((cos(q1).^2.*sin(q2))./2.0+(sin(q1).^2.*sin(q2))./2.0).*2.999511617512276e-1+sin(q1).^2.*(cos(q1).^2+sin(q1).^2).*8.392301883660855e-2+cos(q2+q3).*cos(q1).^2.*cos(q2).*1.499755808756138e-1+cos(q2+q3).*cos(q2).*sin(q1).^2.*1.499755808756138e-1-sin(q2+q3).*cos(q1).^2.*cos(q2).*1.127912389378436e-3-sin(q2+q3).*cos(q2).*sin(q1).^2.*1.127912389378436e-3,cos(q2+q3).*(cos(q1).^2+sin(q1).^2).*8.257807196549019e-4-sin(q2+q3).*(cos(q1).^2+sin(q1).^2).*4.587581372374521e-4,cos(q2+q3).*((cos(q1).^2.*sin(q2))./2.0+(sin(q1).^2.*sin(q2))./2.0).*2.255824778756872e-3+cos(q1).^2.*(cos(q1).^2+sin(q1).^2).*8.392301883660855e-2+sin(q2+q3).*((cos(q1).^2.*sin(q2))./2.0+(sin(q1).^2.*sin(q2))./2.0).*2.999511617512276e-1+sin(q1).^2.*(cos(q1).^2+sin(q1).^2).*8.392301883660855e-2+cos(q2+q3).*cos(q1).^2.*cos(q2).*1.499755808756138e-1+cos(q2+q3).*cos(q2).*sin(q1).^2.*1.499755808756138e-1-sin(q2+q3).*cos(q1).^2.*cos(q2).*1.127912389378436e-3-sin(q2+q3).*cos(q2).*sin(q1).^2.*1.127912389378436e-3,cos(q1).^2.*(cos(q1).^2+sin(q1).^2).*8.392301883660855e-2+sin(q1).^2.*(cos(q1).^2+sin(q1).^2).*8.392301883660855e-2],[3,3]);
